simulink model "sn_high_neg_delta_v25a"  (R2025a)
settings: Solver=VariableStepAuto  StartTime=0.0  StopTime=10.0  RelTol=1e-3
settings Model: Creator=jdcjd  LastModifiedBy=jdcjd

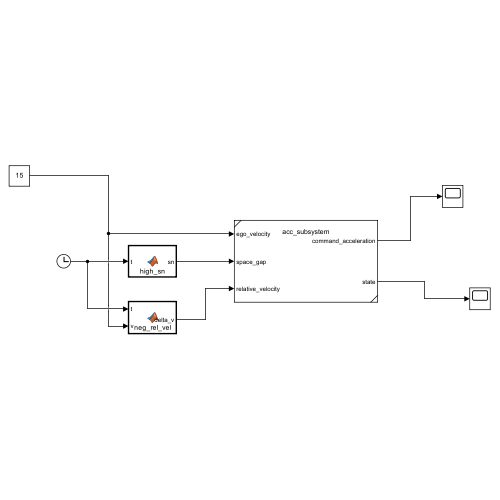
[thumbnail: Simulink's stored preview of the top-level diagram]
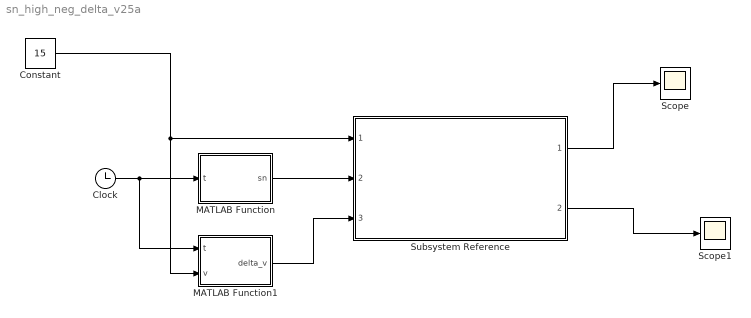
== system sn_high_neg_delta_v25a ==
  Clock : Clock
  Constant : Constant  Value=15
  MATLAB Function : MATLAB Function  TreatAsAtomicUnit=on
  MATLAB Function1 : MATLAB Function  TreatAsAtomicUnit=on
  Scope : Scope
  Scope1 : Scope
  Subsystem Reference : Subsystem  ReferencedSubsystem=acc_subsystem
  wires:
  Clock/1 -> MATLAB Function1/1(t), MATLAB Function/1(t)
  MATLAB Function/1(sn) -> Subsystem Reference/2
  MATLAB Function1/1(delta_v) -> Subsystem Reference/3
  Constant/1 -> Subsystem Reference/1, MATLAB Function1/2(v)
  Subsystem Reference/2 -> Scope1/1
  Subsystem Reference/1 -> Scope/1

== matlab function sn_high_neg_delta_v25a/MATLAB Function ==
  data: t input; sn output
function sn = high_sn(t)

sn = 10 + 5*t;
end

== matlab function sn_high_neg_delta_v25a/MATLAB Function1 ==
  data: t input; delta_v output; v input
function delta_v = neg_rel_vel(t, v)

delta_v = -abs(3 * t -v);
